simulink model "ex"  (R2018a)
settings: Solver=VariableStepAuto  StartTime=0.0  StopTime=10.0  RelTol=1e-3
values from neighbouring files (symbols this model uses):
  d = 0.0445    [DDMRsimulinkParameters.m]    (also in Params.m = 1; dataSimulink.mat; p3dx_constants.m = 0.381)
  J = M*1.2e-1    (= 1.08)    [DDMRsimulinkParameters.m]    (also in Params.m = 1; dataSimulink.mat = 0.192; p3dx_constants.m = 0.2641395)
  Kb = 0.023    [DDMRsimulinkParameters.m]    (also in Params.m = 1; dataSimulink.mat = 0.029; p3dx_constants.m = 0.08)
  Kt = 0.029    [DDMRsimulinkParameters.m]    (also in Params.m = 1; dataSimulink.mat = 0.023; p3dx_constants.m = 0.01)
  L = 0.1655    [DDMRsimulinkParameters.m]    (also in Params.m = 1; dataSimulink.mat; p3dx_constants.m = 0.381)
  La = 0.66e-3    (= 0.00066)    [DDMRsimulinkParameters.m]    (also in Params.m = 1; dataSimulink.mat; p3dx_constants.m = 0.1)
  M = 9    [DDMRsimulinkParameters.m]    (also in Params.m = 1; dataSimulink.mat = 1.6; p3dx_constants.m)
  N = 38.3    [DDMRsimulinkParameters.m]    (also in Params.m = 1; dataSimulink.mat = 1; p3dx_constants.m = 38.1)
  R = 195e-3/2    (= 0.0975)    [DDMRsimulinkParameters.m]    (also in Params.m = 1; dataSimulink.mat = 0.097541; p3dx_constants.m)
  Ra = 0.71    [DDMRsimulinkParameters.m]    (also in Params.m = 1; dataSimulink.mat; p3dx_constants.m = 1)
settings Model: Creator=Egydio Tadeu  LastModifiedBy=Egydio Tadeu

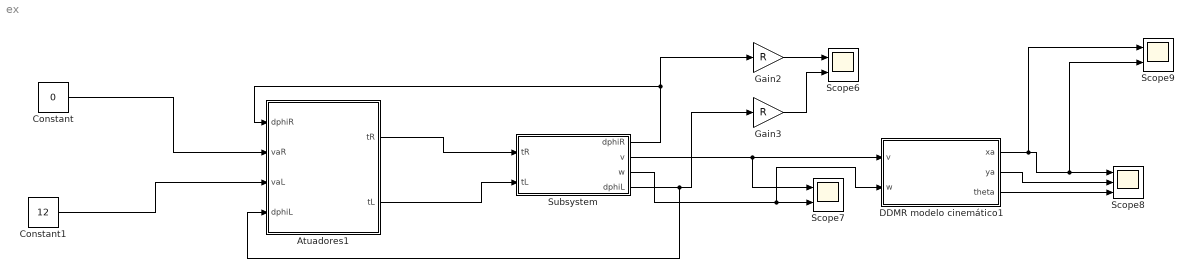
== system ex ==
  Atuadores1 : Subsystem
  Constant : Constant  Value=0
  Constant1 : Constant  Value=12
  DDMR modelo cinemático1 : Subsystem
  Gain2 : Gain  Gain=R
  Gain3 : Gain  Gain=R
  Scope6 : Scope  NumInputPorts=2
  Scope7 : Scope  NumInputPorts=2
  Scope8 : Scope  NumInputPorts=3
  Scope9 : Scope  NumInputPorts=2
  Subsystem : Subsystem
  wires:
  Atuadores1/1(tR) -> Subsystem/1(tR)
  Subsystem/1(dphiR) -> Atuadores1/1(dphiR), Gain2/1
  Subsystem/2(v) -> DDMR modelo cinemático1/1(v), Scope7/1
  Gain3/1 -> Scope6/2
  Gain2/1 -> Scope6/1
  DDMR modelo cinemático1/1(xa) -> Scope9/1, Scope9/2, Scope8/1
  DDMR modelo cinemático1/2(ya) -> Scope8/2
  DDMR modelo cinemático1/3(theta) -> Scope8/3
  Subsystem/3(w) -> DDMR modelo cinemático1/2(w), Scope7/2
  Subsystem/4(dphiL) -> Atuadores1/4(dphiL), Gain3/1
  Atuadores1/2(tL) -> Subsystem/2(tL)
  Constant1/1 -> Atuadores1/3(vaL)
  Constant/1 -> Atuadores1/2(vaR)

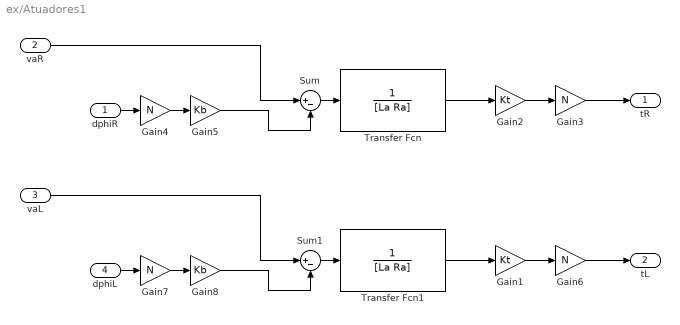
== system ex/Atuadores1 ==
  dphiR : Inport
  vaR : Inport  Port=2
  vaL : Inport  Port=3
  dphiL : Inport  Port=4
  Gain1 : Gain  Gain=Kt
  Gain2 : Gain  Gain=Kt
  Gain{3..4,6..7} (4 alike) : Gain  Gain=N
  Gain5 : Gain  Gain=Kb
  Gain8 : Gain  Gain=Kb
  Sum : Sum  Inputs=|+-
  Sum1 : Sum  Inputs=|+-
  Transfer Fcn : TransferFcn  Denominator=[La Ra]
  Transfer Fcn1 : TransferFcn  Denominator=[La Ra]
  tR : Outport
  tL : Outport  Port=2
  wires:
  Gain3/1 -> tR/1
  Transfer Fcn/1 -> Gain2/1
  Gain2/1 -> Gain3/1
  vaR/1 -> Sum/1
  Gain4/1 -> Gain5/1
  dphiR/1 -> Gain4/1
  Gain5/1 -> Sum/2
  dphiL/1 -> Gain7/1
  Gain6/1 -> tL/1
  Gain1/1 -> Gain6/1
  Transfer Fcn1/1 -> Gain1/1
  Gain7/1 -> Gain8/1
  Gain8/1 -> Sum1/2
  Sum/1 -> Transfer Fcn/1
  Sum1/1 -> Transfer Fcn1/1
  vaL/1 -> Sum1/1

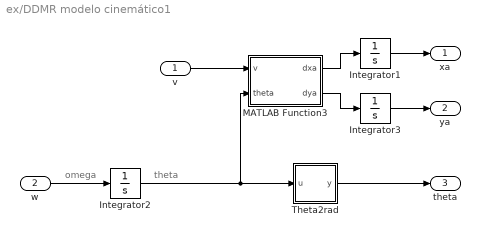
== system ex/DDMR modelo cinemático1 ==
  note: theta
  note: omega
  v : Inport
  w : Inport  Port=2
  Integrator1 : Integrator
  Integrator2 : Integrator
  Integrator3 : Integrator
  MATLAB Function3 : MATLAB Function  TreatAsAtomicUnit=on
  Theta2rad : MATLAB Function  TreatAsAtomicUnit=on
  xa : Outport
  ya : Outport  Port=2
  theta : Outport  Port=3
  wires:
  w/1 -> Integrator2/1
  v/1 -> MATLAB Function3/1(v)
  MATLAB Function3/1(dxa) -> Integrator1/1
  MATLAB Function3/2(dya) -> Integrator3/1
  Integrator1/1 -> xa/1
  Integrator3/1 -> ya/1
  Integrator2/1 -> MATLAB Function3/2(theta), Theta2rad/1(u)
  Theta2rad/1(y) -> theta/1

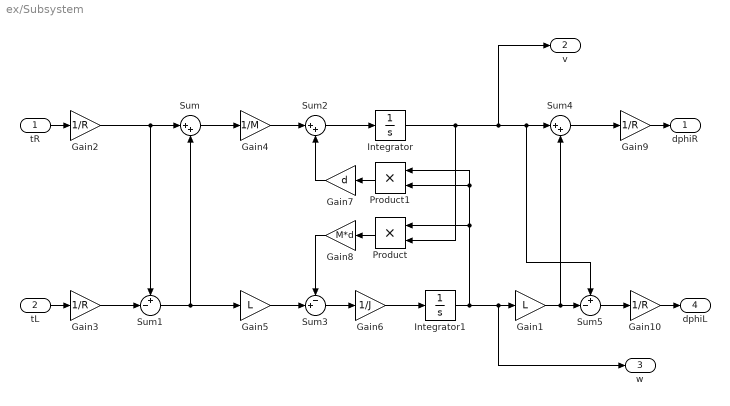
== system ex/Subsystem ==
  tR : Inport
  tL : Inport  Port=2
  Gain1 : Gain  Gain=L
  Gain{2..3,9..10} (4 alike) : Gain  Gain=1/R
  Gain4 : Gain  Gain=1/M
  Gain5 : Gain  Gain=L
  Gain6 : Gain  Gain=1/J
  Gain7 : Gain  Gain=d
  Gain8 : Gain  Gain=M*d
  Integrator : Integrator
  Integrator1 : Integrator
  Product : Product
  Product1 : Product
  Sum : Sum  Inputs=|++
  Sum1 : Sum  Inputs=+-|
  Sum2 : Sum  Inputs=|++
  Sum3 : Sum  Inputs=-+|
  Sum4 : Sum  Inputs=|++
  Sum5 : Sum  Inputs=+-|
  dphiR : Outport
  v : Outport  Port=2
  w : Outport  Port=3
  dphiL : Outport  Port=4
  wires:
  Gain8/1 -> Sum3/1
  tL/1 -> Gain3/1
  Sum4/1 -> Gain9/1
  Sum2/1 -> Integrator/1
  Product1/1 -> Gain7/1
  Gain10/1 -> dphiL/1
  Sum5/1 -> Gain10/1
  Gain2/1 -> Sum1/1, Sum/1
  Product/1 -> Gain8/1
  Integrator1/1 -> w/1, Gain1/1, Product/1, Product1/1, Product1/2
  Gain4/1 -> Sum2/1
  Gain3/1 -> Sum1/2
  Gain5/1 -> Sum3/2
  Sum/1 -> Gain4/1
  Sum1/1 -> Sum/2, Gain5/1
  Gain7/1 -> Sum2/2
  Integrator/1 -> Product/2, v/1, Sum4/1, Sum5/1
  Sum3/1 -> Gain6/1
  Gain6/1 -> Integrator1/1
  tR/1 -> Gain2/1
  Gain9/1 -> dphiR/1
  Gain1/1 -> Sum4/2, Sum5/2

== matlab function ex/DDMR modelo cinemático1/MATLAB Function3 ==
  data: v input; dxa output; theta input; dya output
function [dxa, dya]  = fcn(v, theta)

dxa = cos(theta)*v;
dya = sin(theta)*v;

== matlab function ex/DDMR modelo cinemático1/Theta2rad ==
  data: u input; y output
function y = fcn(u)

y = u;
while (abs(y) > pi)
    if(y > 0)
        y = y - 2*pi;
    else
        y = y + 2*pi;
    end
end

end
